simulink model "example1"  (R2019b)
settings: Solver=ode45  StartTime=0.0  StopTime=3  FixedStep=100  RelTol=1e-3  AbsTol=1e-6
settings Model: Creator=davis  LastModifiedBy=davis

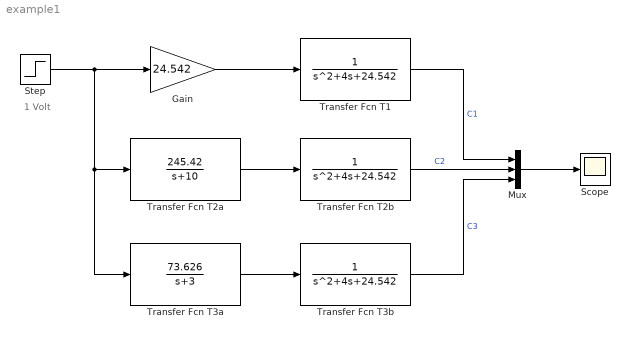
== system example1 ==
  note: 1 Volt
  Gain : Gain  Gain=24.542
  Mux : Mux  Inputs=3
  Scope : Scope
  Step : Step  Time=0  SampleTime=0
  Transfer Fcn T1 : TransferFcn  Denominator=[1 4 24.542]
  Transfer Fcn T2a : TransferFcn  Numerator=[245.42]  Denominator=[1 10]
  Transfer Fcn T2b : TransferFcn  Denominator=[1 4 24.542]
  Transfer Fcn T3a : TransferFcn  Numerator=[73.626]  Denominator=[1 3]
  Transfer Fcn T3b : TransferFcn  Denominator=[1 4 24.542]
  wires:
  Step/1 -> Transfer Fcn T2a/1, Transfer Fcn T3a/1, Gain/1
  Transfer Fcn T2b/1 -> Mux/2  "C2"
  Transfer Fcn T1/1 -> Mux/1  "C1"
  Transfer Fcn T3b/1 -> Mux/3  "C3"
  Gain/1 -> Transfer Fcn T1/1
  Transfer Fcn T2a/1 -> Transfer Fcn T2b/1
  Transfer Fcn T3a/1 -> Transfer Fcn T3b/1
  Mux/1 -> Scope/1
